simulink library "starslibKinematicalEquations"  (R2024b)
settings: Solver=ode45  StartTime=0.0  StopTime=10.0  RelTol=1e-3  EnableMultiTasking=on
libraries: starslibAxisTransformations x6, starslibMathOperations x5, $bdroot x1
settings Model: Creator=eheim  LastModifiedBy=gryph
settings SolverCC: AlgebraicLoopSolver=TrustRegion
settings DataIOCC: LimitDataPoints=on  SaveFormat=Array  SignalLoggingSaveFormat=ModelDataLogs  ReturnWorkspaceOutputs=off
settings OptimizationCC: ReuseModelBlockBuffer=off  ExpressionDepthLimit=2147483647  LifeSpan=inf
settings DebuggingCC: UnderspecifiedInitializationDetection=Classic  MergeDetectMultiDrivingBlocksExec=none  SolverPrmCheckMsg=warning  FcnCallInpInsideContextMsg=warning  UnconnectedInputMsg=warning  UnconnectedOutputMsg=warning  UnconnectedLineMsg=warning  StateNameClashWarn=warning  SFUnexpectedBacktrackingDiag=warning  SFNoUnconditionalDefaultTransitionDiag=warning  SFExecutionAtInitializationDiag=none  ArithmeticOperatorsInVariantConditions=warning
settings HardwareCC: ProdBitPerPointer=32  ProdBitPerSizeT=32  ProdBitPerPtrDiffT=32  ProdLargestAtomicFloat=None  ProdIntDivRoundTo=Undefined  ProdEndianess=Unspecified  ProdWordSize=32  ProdHWDeviceType=32-bit Generic
settings ModelReferenceCC: PropagateSignalLabelsOutOfModel=off
settings SFSimCC: SimUseLocalCustomCode=off  CustomCodeUndefinedFunction=UseInterfaceOnly
settings RTWCC: RTWUseLocalCustomCode=off  GPUComputeCapability=3.5
settings CodeAppCC: StateflowObjectComments=on
settings GRTTargetCC: TargetLangStandard=C89/C90 (ANSI)  CombineOutputUpdateFcns=off  GRTInterface=on
settings ConfigComp: CovMetricSettings=dw  CovSaveCumulativeToWorkspaceVar=on  CovSaveSingleToWorkspaceVar=on  CovExternalEMLEnable=off  CovSFcnEnable=off

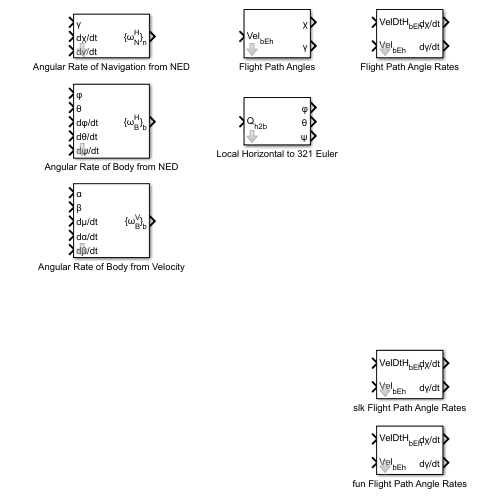
[thumbnail: Simulink's stored preview of the top-level diagram]
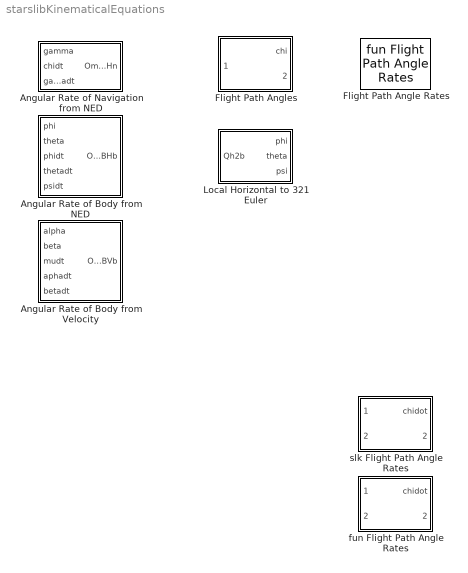
== system starslibKinematicalEquations ==
  Angular Rate of Body from NED : Subsystem  mask(Angular Rate of Body from NED){}
      mask help: Given 3-2-1 Euler angles in radians and their angular rates this block computes the angular rate of the body frame relative to the angular rate of the NED frame in radians persecond and expressed in body coordinates.
      mask Display:
      | port_label('input' ,1,'\phi','texmode','on')
      | port_label('input' ,2,'\theta','texmode','on')
      | port_label('input' ,3,'d\phi/dt','texmode','on')
      | port_label('input' ,4,'d\theta/dt','texmode','on')
      | port_label('input' ,5,'d\psi/dt','texmode','on')
      | port_label('output',1,'\{\omega_B^H\}_b','texmode','on')
  Angular Rate of Body from Velocity : Subsystem  mask(Angular Rate of Body from Velocity){}
      mask help: Given mu, beta, alpha in radians and their angular rates this block computes the angular rate of the body frame relative to the angular rate of the velocity frame in radians per second and expressed in body coordinates.
      mask Display:
      | port_label('input' ,1,'\alpha','texmode','on')
      | port_label('input' ,2,'\beta','texmode','on')
      | port_label('input' ,3,'d\mu/dt','texmode','on')
      | port_label('input' ,4,'d\alpha/dt','texmode','on')
      | port_label('input' ,5,'d\beta/dt','texmode','on')
      | port_label('output',1,'\{\omega_B^V\}_b','texmode','on')
  Angular Rate of Navigation from NED : Subsystem  mask(Angular Rate of Navigation from NED){}
      mask help: Given flight path angle and ground track angles in radians and their angular rates this block computes the angular rate of the navigation frame relative to the angular rate of the NED frame in radians persecond and expressed in navigation coordinates.
      mask Display:
      | port_label('input' ,1,'\gamma','texmode','on')
      | port_label('input' ,2,'d\chi/dt','texmode','on')
      | port_label('input' ,3,'d\gamma/dt','texmode','on')
      | port_label('output',1,'\{\omega_N^H\}_n','texmode','on')
  Flight Path Angle Rates : $bdroot/fun Flight Path Angle Rates
  Flight Path Angles : Subsystem  mask(Flight Path Angles){}
      mask help: Computes flight path angle, gamma and ground track angle, chi. Inputs must be in the local North East Down (NED) coordinate system and relative to the rotating world.
      mask Display:
      | port_label('input' ,1,'Vel_{bEh}','texmode','on')
      | port_label('output',1,'\chi','texmode','on')
      | port_label('output',2,'\gamma','texmode','on')
  Local Horizontal to 321 Euler : Subsystem  mask(Local Horizontal to Body Quaternion to 321 Eular Angles){}
      mask help: Converts local vertical local horizontal to body axes quaternion to 3-2-1 Euler bank, attitude and heading angles.
      mask Display:
      | port_label('input',1,'Q_{h2b}','texmode','on')
      | port_label('output',1,'\phi','texmode','on')
      | port_label('output',2,'\theta','texmode','on')
      | port_label('output',3,'\psi','texmode','on')
  fun Flight Path Angle Rates : Subsystem  mask(Flight Path Angle Rates){}
      mask help: Computes time rate of change of flight path angle gamma and ground track angle chi. Inputs must be in the local North East Down (NED) coordinate system and relative to the rotating world. Note acceleration of the NED frame must subtract the angular rate of NED frame (relative to the rotating world) cross the velocity of the NED frame relative to the rotating world, i.e. AccelE_h - Omegah_h x VelE_h.
      mask Display:
      | port_label('input' ,1,'VelDtH_{bEh}','texmode','on')
      | port_label('input' ,2,'Vel_{bEh}','texmode','on')
      | port_label('output',2,'d\gamma/dt','texmode','on')
      | port_label('output',1,'d\chi/dt','texmode','on')
  slk Flight Path Angle Rates : Subsystem  mask(Flight Path Angle Rates){}
      mask help: Computes time rate of change of flight path angle gamma and ground track angle chi. Inputs must be in the local North East Down (NED) coordinate system and relative to the rotating world. Note acceleration of the NED frame must subtract the angular rate of NED frame (relative to the rotating world) cross the velocity of the NED frame relative to the rotating world, i.e. AccelE_h - Omegah_h x VelE_h.
      mask Display:
      | port_label('input' ,1,'VelDtH_{bEh}','texmode','on')
      | port_label('input' ,2,'Vel_{bEh}','texmode','on')
      | port_label('output',2,'d\gamma/dt','texmode','on')
      | port_label('output',1,'d\chi/dt','texmode','on')

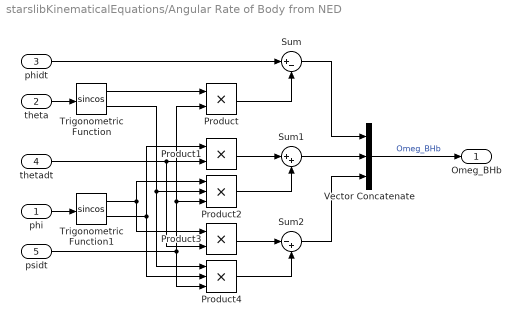
== system starslibKinematicalEquations/Angular Rate of Body from NED ==
  phi : Inport
  theta : Inport  Port=2
  phidt : Inport  Port=3
  thetadt : Inport  Port=4
  psidt : Inport  Port=5
  Product : Product  RndMeth=Zero
  Product1 : Product  RndMeth=Zero
  Product2 : Product  Inputs=3  RndMeth=Zero
  Product3 : Product  RndMeth=Zero
  Product4 : Product  Inputs=3  RndMeth=Zero
  Sum : Sum  Inputs=|+-
  Sum1 : Sum  Inputs=|++
  Sum2 : Sum  Inputs=|-+
  Trigonometric Function : Trigonometry  Operator=sincos
  Trigonometric Function1 : Trigonometry  Operator=sincos
  Vector Concatenate : Concatenate  NumInputs=3  Mode=Multidimensional array
  Omeg_BHb : Outport
  wires:
  Sum2/1 -> Vector Concatenate/3
  Sum1/1 -> Vector Concatenate/2
  Sum/1 -> Vector Concatenate/1
  Trigonometric Function1/1 -> Product3/1, Product2/1
  Trigonometric Function1/2 -> Product1/1, Product4/2
  Trigonometric Function/2 -> Product2/2, Product4/1
  thetadt/1 -> Product3/2, Product1/2
  psidt/1 -> Product/2, Product2/3, Product4/3
  phidt/1 -> Sum/1
  Product/1 -> Sum/2
  Trigonometric Function/1 -> Product/1
  Product4/1 -> Sum2/2
  Product3/1 -> Sum2/1
  Product2/1 -> Sum1/2
  Product1/1 -> Sum1/1
  phi/1 -> Trigonometric Function1/1
  theta/1 -> Trigonometric Function/1
  Vector Concatenate/1 -> Omeg_BHb/1  "Omeg_BHb"

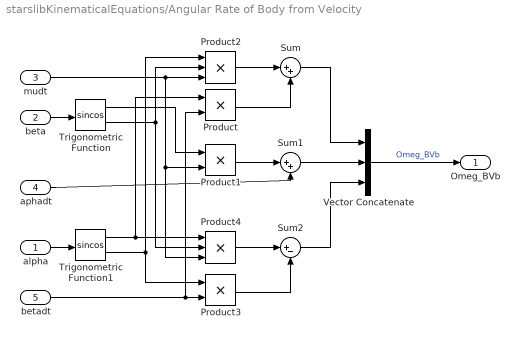
== system starslibKinematicalEquations/Angular Rate of Body from Velocity ==
  alpha : Inport
  beta : Inport  Port=2
  mudt : Inport  Port=3
  aphadt : Inport  Port=4
  betadt : Inport  Port=5
  Product : Product  RndMeth=Zero
  Product1 : Product  RndMeth=Zero
  Product2 : Product  Inputs=3  RndMeth=Zero
  Product3 : Product  RndMeth=Zero
  Product4 : Product  Inputs=3  RndMeth=Zero
  Sum : Sum  Inputs=|++
  Sum1 : Sum  Inputs=|++
  Sum2 : Sum  Inputs=|+-
  Trigonometric Function : Trigonometry  Operator=sincos
  Trigonometric Function1 : Trigonometry  Operator=sincos
  Vector Concatenate : Concatenate  NumInputs=3  Mode=Multidimensional array
  Omeg_BVb : Outport
  wires:
  Product3/1 -> Sum2/2
  betadt/1 -> Product3/2, Product/2
  Trigonometric Function1/2 -> Product3/1, Product2/1
  Trigonometric Function1/1 -> Product/1, Product4/1
  Trigonometric Function/2 -> Product4/2, Product2/2
  Product4/1 -> Sum2/1
  mudt/1 -> Product4/3, Product1/2, Product2/3
  Trigonometric Function/1 -> Product1/1
  aphadt/1 -> Sum1/2
  Product1/1 -> Sum1/1
  Product2/1 -> Sum/1
  Product/1 -> Sum/2
  Vector Concatenate/1 -> Omeg_BVb/1  "Omeg_BVb"
  beta/1 -> Trigonometric Function/1
  alpha/1 -> Trigonometric Function1/1
  Sum/1 -> Vector Concatenate/1
  Sum1/1 -> Vector Concatenate/2
  Sum2/1 -> Vector Concatenate/3

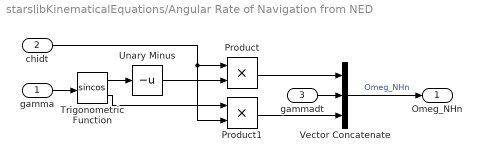
== system starslibKinematicalEquations/Angular Rate of Navigation from NED ==
  gamma : Inport
  chidt : Inport  Port=2
  gammadt : Inport  Port=3
  Product : Product  RndMeth=Zero
  Product1 : Product  RndMeth=Zero
  Trigonometric Function : Trigonometry  Operator=sincos
  Unary Minus : UnaryMinus
  Vector Concatenate : Concatenate  NumInputs=3  Mode=Multidimensional array
  Omeg_NHn : Outport
  wires:
  Trigonometric Function/1 -> Unary Minus/1
  Trigonometric Function/2 -> Product1/1
  Unary Minus/1 -> Product/2
  Product/1 -> Vector Concatenate/1
  Product1/1 -> Vector Concatenate/3
  chidt/1 -> Product/1, Product1/2
  gamma/1 -> Trigonometric Function/1
  gammadt/1 -> Vector Concatenate/2
  Vector Concatenate/1 -> Omeg_NHn/1  "Omeg_NHn"

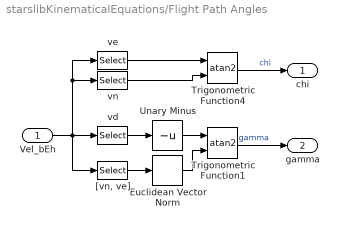
== system starslibKinematicalEquations/Flight Path Angles ==
  Vel_bEh : Inport
  Euclidean Vector Norm : starslibMathOperations/Euclidean Vector Norm  dim=1
  Trigonometric Function1 : Trigonometry  Operator=atan2  OutputSignalType=real
  Trigonometric Function4 : Trigonometry  Operator=atan2  OutputSignalType=real
  Unary Minus : UnaryMinus
  "[vn, ve]" : Selector  NumberOfDimensions=2  InputPortWidth=3  IndexOptions=Index vector (dialog),Select all  Indices=[1 2],1  OutputSizes=1,1
  vd : Selector  NumberOfDimensions=2  InputPortWidth=3  IndexOptions=Index vector (dialog),Select all  Indices=3,1  OutputSizes=1,1
  ve : Selector  NumberOfDimensions=2  InputPortWidth=3  IndexOptions=Index vector (dialog),Select all  Indices=2,1  OutputSizes=1,1
  vn : Selector  NumberOfDimensions=2  InputPortWidth=3  IndexOptions=Index vector (dialog),Select all  Indices=1,1  OutputSizes=1,1
  chi : Outport
  gamma : Outport  Port=2
  wires:
  Vel_bEh/1 -> vd/1, vn/1, ve/1, "[vn, ve]"/1
  vd/1 -> Unary Minus/1
  ve/1 -> Trigonometric Function4/1
  vn/1 -> Trigonometric Function4/2
  Trigonometric Function4/1 -> chi/1  "chi"
  Trigonometric Function1/1 -> gamma/1  "gamma"
  "[vn, ve]"/1 -> Euclidean Vector Norm/1
  Unary Minus/1 -> Trigonometric Function1/1
  Euclidean Vector Norm/1 -> Trigonometric Function1/2

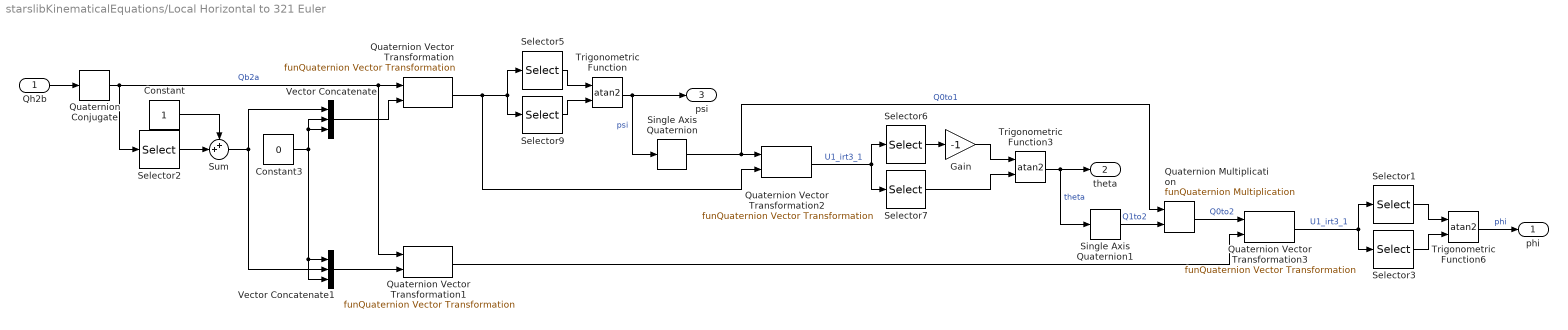
== system starslibKinematicalEquations/Local Horizontal to 321 Euler ==
  Qh2b : Inport
  Constant : Constant
  Constant3 : Constant  Value=0
  Gain : Gain  Gain=-1
  Quaternion Conjugate : starslibMathOperations/Quaternion Conjugate  n=0
  Quaternion Multiplication : starslibMathOperations/funQuaternion Multiplication  n=0
  Quaternion Vector Transformation{,1..3} (4 alike) : starslibAxisTransformations/funQuaternion Vector Transformation  n=0
  Selector1 : Selector  InputPortWidth=3  IndexOptions=Index vector (dialog)  Indices=3  OutputSizes=1
  Selector2 : Selector  InputPortWidth=4  IndexOptions=Index vector (dialog)  Indices=1  OutputSizes=1
  Selector3 : Selector  InputPortWidth=3  IndexOptions=Index vector (dialog)  Indices=2  OutputSizes=1
  Selector5 : Selector  InputPortWidth=3  IndexOptions=Index vector (dialog)  Indices=2  OutputSizes=1
  Selector6 : Selector  InputPortWidth=3  IndexOptions=Index vector (dialog)  Indices=3  OutputSizes=1
  Selector7 : Selector  InputPortWidth=3  IndexOptions=Index vector (dialog)  Indices=1  OutputSizes=1
  Selector9 : Selector  InputPortWidth=3  IndexOptions=Index vector (dialog)  Indices=1  OutputSizes=1
  Single Axis Quaternion : starslibAxisTransformations/Single Axis Quaternion  RotAxis=z  n=0
  Single Axis Quaternion1 : starslibAxisTransformations/Single Axis Quaternion  RotAxis=y  n=0
  Sum : Sum  Inputs=++|
  Trigonometric Function : Trigonometry  Operator=atan2
  Trigonometric Function3 : Trigonometry  Operator=atan2
  Trigonometric Function6 : Trigonometry  Operator=atan2
  Vector Concatenate : Concatenate  NumInputs=3  Mode=Multidimensional array
  Vector Concatenate1 : Concatenate  NumInputs=3  Mode=Multidimensional array
  phi : Outport
  theta : Outport  Port=2
  psi : Outport  Port=3
  wires:
  Quaternion Conjugate/1 -> Quaternion Vector Transformation/1, Quaternion Vector Transformation1/1, Selector2/1  "Qb2a"
  Quaternion Vector Transformation/1 -> Selector5/1, Selector9/1, Quaternion Vector Transformation2/2
  Trigonometric Function/1 -> psi/1, Single Axis Quaternion/1  "psi"
  Single Axis Quaternion/1 -> Quaternion Multiplication/1, Quaternion Vector Transformation2/1  "Q0to1"
  Quaternion Vector Transformation2/1 -> Selector6/1, Selector7/1  "U1_irt3_1"
  Quaternion Vector Transformation1/1 -> Quaternion Vector Transformation3/2
  Trigonometric Function3/1 -> theta/1, Single Axis Quaternion1/1  "theta"
  Single Axis Quaternion1/1 -> Quaternion Multiplication/2  "Q1to2"
  Quaternion Multiplication/1 -> Quaternion Vector Transformation3/1  "Q0to2"
  Quaternion Vector Transformation3/1 -> Selector1/1, Selector3/1  "U1_irt3_1"
  Trigonometric Function6/1 -> phi/1  "phi"
  Qh2b/1 -> Quaternion Conjugate/1
  Constant/1 -> Sum/1
  Selector2/1 -> Sum/2
  Sum/1 -> Vector Concatenate/1, Vector Concatenate1/2
  Selector5/1 -> Trigonometric Function/1
  Selector9/1 -> Trigonometric Function/2
  Vector Concatenate1/1 -> Quaternion Vector Transformation1/2
  Vector Concatenate/1 -> Quaternion Vector Transformation/2
  Constant3/1 -> Vector Concatenate/2, Vector Concatenate/3, Vector Concatenate1/1, Vector Concatenate1/3
  Selector1/1 -> Trigonometric Function6/1
  Selector3/1 -> Trigonometric Function6/2
  Selector6/1 -> Gain/1
  Selector7/1 -> Trigonometric Function3/2
  Gain/1 -> Trigonometric Function3/1

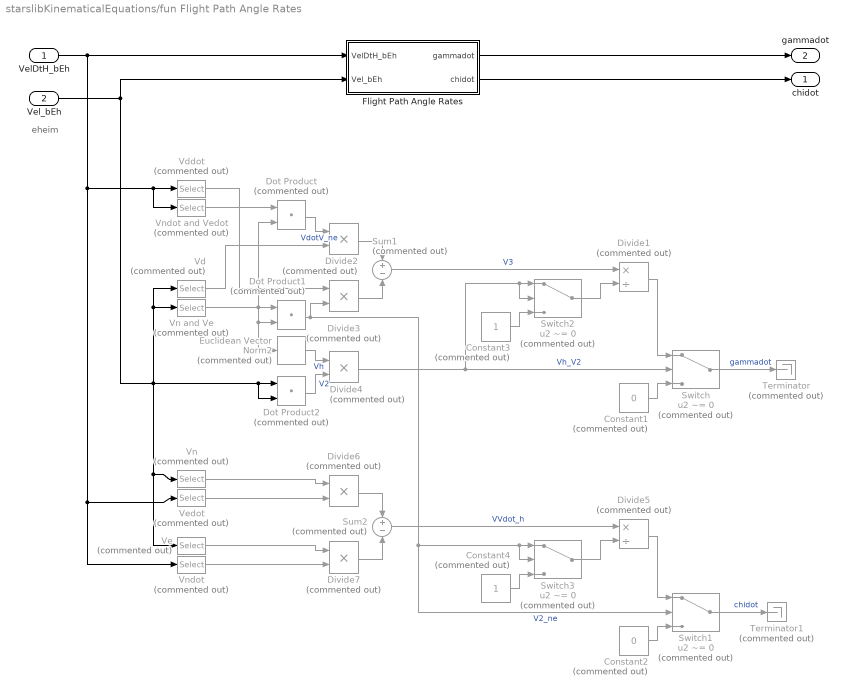
== system starslibKinematicalEquations/fun Flight Path Angle Rates ==
  note: eheim
  VelDtH_bEh : Inport
  Vel_bEh : Inport  Port=2
  Constant1 : Constant  Commented=on  Value=0
  Constant2 : Constant  Commented=on  Value=0
  Constant3 : Constant  Commented=on
  Constant4 : Constant  Commented=on
  Divide1 : Product  Commented=on  Inputs=*/
  Divide{2..4,6..7} (5 alike) : Product  Commented=on
  Divide5 : Product  Commented=on  Inputs=*/
  Dot Product : DotProduct  Commented=on  OutDataTypeStr=Inherit: Inherit via internal rule
  Dot Product1 : DotProduct  Commented=on  OutDataTypeStr=Inherit: Inherit via internal rule
  Dot Product2 : DotProduct  Commented=on  OutDataTypeStr=Inherit: Inherit via internal rule
  Euclidean Vector Norm2 : starslibMathOperations/Euclidean Vector Norm  Commented=on  dim=1
  Flight Path Angle Rates : MATLAB Function  TreatAsAtomicUnit=on
  Sum1 : Sum  Commented=on  Inputs=+|-
  Sum2 : Sum  Commented=on  Inputs=+|-
  Switch{,1..3} (4 alike) : Switch  Commented=on  Criteria=u2 ~= 0  SaturateOnIntegerOverflow=off  InputSameDT=off
  Terminator : Terminator  Commented=on
  Terminator1 : Terminator  Commented=on
  Vd : Selector  Commented=on  NumberOfDimensions=2  InputPortWidth=3  IndexOptions=Index vector (dialog),Select all  Indices=3,1  OutputSizes=1,1
  Vddot : Selector  Commented=on  NumberOfDimensions=2  InputPortWidth=3  IndexOptions=Index vector (dialog),Select all  Indices=3,1  OutputSizes=1,1
  Ve : Selector  Commented=on  NumberOfDimensions=2  InputPortWidth=3  IndexOptions=Index vector (dialog),Select all  Indices=2,1  OutputSizes=1,1
  Vedot : Selector  Commented=on  NumberOfDimensions=2  InputPortWidth=3  IndexOptions=Index vector (dialog),Select all  Indices=2,1  OutputSizes=1,1
  Vn : Selector  Commented=on  NumberOfDimensions=2  InputPortWidth=3  IndexOptions=Index vector (dialog),Select all  Indices=1,1  OutputSizes=1,1
  Vn and Ve : Selector  Commented=on  NumberOfDimensions=2  InputPortWidth=3  IndexOptions=Index vector (dialog),Select all  Indices=[1 2],1  OutputSizes=1,1
  Vndot : Selector  Commented=on  NumberOfDimensions=2  InputPortWidth=3  IndexOptions=Index vector (dialog),Select all  Indices=1,1  OutputSizes=1,1
  Vndot and Vedot : Selector  Commented=on  NumberOfDimensions=2  InputPortWidth=3  IndexOptions=Index vector (dialog),Select all  Indices=[1 2],1  OutputSizes=1,1
  chidot : Outport
  gammadot : Outport  Port=2
  wires:
  Constant4/1 -> Switch3/3
  Switch3/1 -> Divide5/2
  Switch2/1 -> Divide1/2
  Constant3/1 -> Switch2/3
  VelDtH_bEh/1 -> Flight Path Angle Rates/1(VelDtH_bEh), Vndot/1, Vedot/1, Vndot and Vedot/1, Vddot/1
  Vndot and Vedot/1 -> Dot Product/1
  Vn and Ve/1 -> Dot Product1/1, Dot Product/2, Dot Product1/2, Euclidean Vector Norm2/1
  Vd/1 -> Divide2/2
  Dot Product/1 -> Divide2/1  "VdotV_ne"
  Vddot/1 -> Divide3/1
  Dot Product1/1 -> Divide3/2, Switch3/1, Switch3/2, Switch1/2  "V2_ne"
  Divide2/1 -> Sum1/1
  Divide3/1 -> Sum1/2
  Sum1/1 -> Divide1/1  "V3"
  Dot Product2/1 -> Divide4/2  "V2"
  Divide4/1 -> Switch/2, Switch2/1, Switch2/2  "Vh_V2"
  Constant1/1 -> Switch/3
  Divide1/1 -> Switch/1
  Euclidean Vector Norm2/1 -> Divide4/1  "Vh"
  Divide6/1 -> Sum2/1
  Divide7/1 -> Sum2/2
  Sum2/1 -> Divide5/1  "VVdot_h"
  Constant2/1 -> Switch1/3
  Divide5/1 -> Switch1/1
  Vn/1 -> Divide6/1
  Vedot/1 -> Divide6/2
  Ve/1 -> Divide7/1
  Vndot/1 -> Divide7/2
  Vel_bEh/1 -> Flight Path Angle Rates/2(Vel_bEh), Vd/1, Vn and Ve/1, Dot Product2/1, Dot Product2/2, Vn/1, Ve/1
  Switch/1 -> Terminator/1  "gammadot"
  Switch1/1 -> Terminator1/1  "chidot"
  Flight Path Angle Rates/1(gammadot) -> gammadot/1
  Flight Path Angle Rates/2(chidot) -> chidot/1

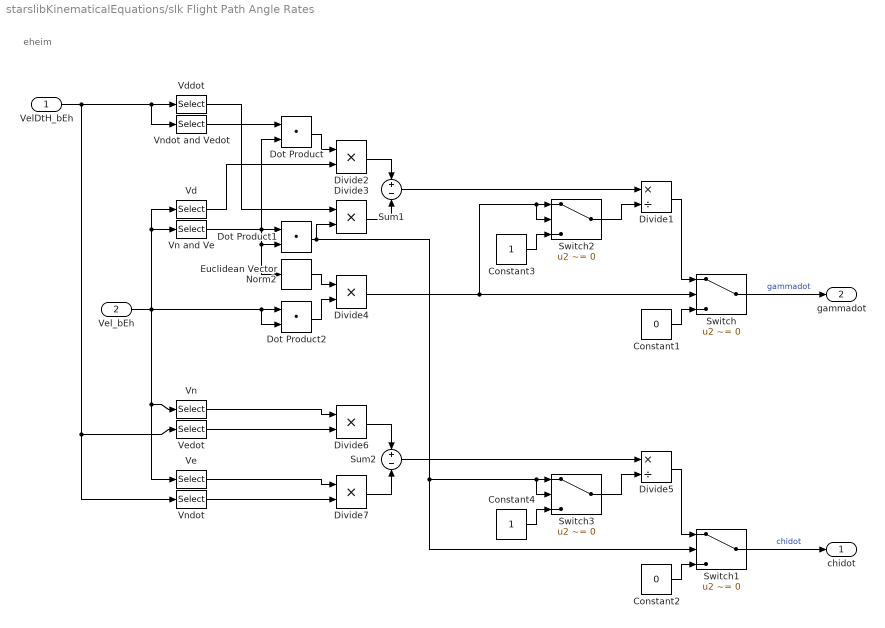
== system starslibKinematicalEquations/slk Flight Path Angle Rates ==
  note: eheim
  VelDtH_bEh : Inport
  Vel_bEh : Inport  Port=2
  Constant1 : Constant  Value=0
  Constant2 : Constant  Value=0
  Constant3 : Constant
  Constant4 : Constant
  Divide1 : Product  Inputs=*/
  Divide{2..4,6..7} (5 alike) : Product
  Divide5 : Product  Inputs=*/
  Dot Product : DotProduct  OutDataTypeStr=Inherit: Inherit via internal rule
  Dot Product1 : DotProduct  OutDataTypeStr=Inherit: Inherit via internal rule
  Dot Product2 : DotProduct  OutDataTypeStr=Inherit: Inherit via internal rule
  Euclidean Vector Norm2 : starslibMathOperations/Euclidean Vector Norm  dim=1
  Sum1 : Sum  Inputs=+|-
  Sum2 : Sum  Inputs=+|-
  Switch{,1..3} (4 alike) : Switch  Criteria=u2 ~= 0  SaturateOnIntegerOverflow=off  InputSameDT=off
  Vd : Selector  NumberOfDimensions=2  InputPortWidth=3  IndexOptions=Index vector (dialog),Select all  Indices=3,1  OutputSizes=1,1
  Vddot : Selector  NumberOfDimensions=2  InputPortWidth=3  IndexOptions=Index vector (dialog),Select all  Indices=3,1  OutputSizes=1,1
  Ve : Selector  NumberOfDimensions=2  InputPortWidth=3  IndexOptions=Index vector (dialog),Select all  Indices=2,1  OutputSizes=1,1
  Vedot : Selector  NumberOfDimensions=2  InputPortWidth=3  IndexOptions=Index vector (dialog),Select all  Indices=2,1  OutputSizes=1,1
  Vn : Selector  NumberOfDimensions=2  InputPortWidth=3  IndexOptions=Index vector (dialog),Select all  Indices=1,1  OutputSizes=1,1
  Vn and Ve : Selector  NumberOfDimensions=2  InputPortWidth=3  IndexOptions=Index vector (dialog),Select all  Indices=[1 2],1  OutputSizes=1,1
  Vndot : Selector  NumberOfDimensions=2  InputPortWidth=3  IndexOptions=Index vector (dialog),Select all  Indices=1,1  OutputSizes=1,1
  Vndot and Vedot : Selector  NumberOfDimensions=2  InputPortWidth=3  IndexOptions=Index vector (dialog),Select all  Indices=[1 2],1  OutputSizes=1,1
  chidot : Outport
  gammadot : Outport  Port=2
  wires:
  Constant4/1 -> Switch3/3
  Switch3/1 -> Divide5/2
  Switch2/1 -> Divide1/2
  Constant3/1 -> Switch2/3
  VelDtH_bEh/1 -> Vndot/1, Vedot/1, Vndot and Vedot/1, Vddot/1
  Vndot and Vedot/1 -> Dot Product/1
  Vn and Ve/1 -> Dot Product1/1, Dot Product/2, Dot Product1/2, Euclidean Vector Norm2/1
  Vd/1 -> Divide2/2
  Dot Product/1 -> Divide2/1
  Vddot/1 -> Divide3/1
  Dot Product1/1 -> Divide3/2, Switch3/1, Switch3/2, Switch1/2
  Divide2/1 -> Sum1/1
  Divide3/1 -> Sum1/2
  Sum1/1 -> Divide1/1
  Dot Product2/1 -> Divide4/2
  Divide4/1 -> Switch/2, Switch2/1, Switch2/2
  Constant1/1 -> Switch/3
  Divide1/1 -> Switch/1
  Euclidean Vector Norm2/1 -> Divide4/1
  Divide6/1 -> Sum2/1
  Divide7/1 -> Sum2/2
  Sum2/1 -> Divide5/1
  Constant2/1 -> Switch1/3
  Divide5/1 -> Switch1/1
  Vn/1 -> Divide6/1
  Vedot/1 -> Divide6/2
  Ve/1 -> Divide7/1
  Vndot/1 -> Divide7/2
  Vel_bEh/1 -> Vd/1, Vn and Ve/1, Dot Product2/1, Dot Product2/2, Vn/1, Ve/1
  Switch/1 -> gammadot/1  "gammadot"
  Switch1/1 -> chidot/1  "chidot"

== matlab function starslibKinematicalEquations/fun Flight Path Angle Rates/Flight Path Angle Rates ==
  data: VelDtH_bEh input; gammadot output; Vel_bEh input; chidot output
function [gammadot, chidot] = fcn(VelDtH_bEh, Vel_bEh)
% Replicates the Simulink blocks computing flight path angle rates in NED


Vndot = VelDtH_bEh(1,:);
Vedot = VelDtH_bEh(2,:);
Vddot = VelDtH_bEh(3,:); 

Vn = Vel_bEh(1,:);
Ve = Vel_bEh(2,:);
Vd = Vel_bEh(3,:); 



VdotV_ne = dot([Vndot; Vedot], [Vn; Ve]);
V2_ne = dot([Vn; Ve], [Vn; Ve]);
V2 = dot(Vel_bEh(1:3,:), Vel_bEh(1:3,:)); % Indices (1:3,:) serve to 'declare' size of vector

Vh_V2 = norm([Vn; Ve], 2) .* V2; % Vh = horizontal velocity
V3 = (VdotV_ne .* Vd) - (Vddot .* V2_ne);

if Vh_V2 ~= 0
    gammadot = V3./Vh_V2;
else
    gammadot = 0;
end

VVdot_h = (Vn .* Vedot) - (Ve .* Vndot);

if V2_ne ~= 0 
    chidot = VVdot_h / V2_ne;
else
    chidot = 0;
end

end
